simulink model "PWM"  (Simulink 7.5)
settings: Solver=VariableStepDiscrete  StartTime=0.0  StopTime=1  MaxStep=0.0001  RelTol=1e-3
libraries: simulink x1, powerlib x1
settings Model: Creator=lm  LastModifiedBy=lm

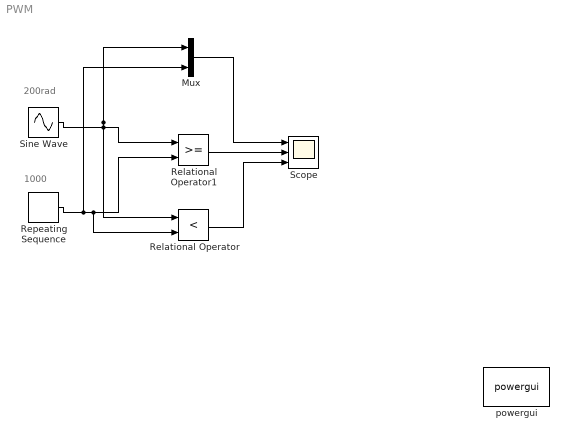
== system PWM ==
  note: 200rad
  note: 1000
  Mux : Mux  Inputs=2
  Relational Operator : RelationalOperator  Operator=<  LogicOutDataTypeMode=boolean  LogicDataType=fixdt(0, 8)  OutDataTypeStr=boolean
  Relational Operator1 : RelationalOperator  LogicOutDataTypeMode=boolean  LogicDataType=fixdt(0, 8)  OutDataTypeStr=boolean
  Repeating Sequence : simulink/Sources/Repeating Sequence  SystemSampleTime=-1  rep_seq_t=[0 0.002]  rep_seq_y=[-1 1]
  Scope : Scope  NumInputPorts=3
      settings: TimeRange=5  YMin=0~-5~-5  YMax=1~5~5
  Sine Wave : Sin  Amplitude=0.8  Bias=0  Frequency=200  Phase=0  Samples=0.02  SampleTime=0  Offset=0
  powergui : powerlib/powergui  Priority=1  SystemSampleTime=-1  SimulationMode=Continuous  SampleTime=50e-6  frequency=60  SPID=off  DisableSnubberDevices=off  DisableRonSwitches=off  DisableVfSwitches=off  SwTol=0  Interpol=off  frequencyindice=60  echomessages=off  HookPort=off  DisplayEquations=off  FunctionMessages=off  EnableUseOfTLC=off  x0status=blocks  RestoreLinks=warning  ResistiveCurrentMeasurement=off  Ylog=off  Xlog=on  ShowGrid=off  save=off  variable=ZData  ZoomFFT=off  StartTime=0.0  cycles=1  DisplayStyle=1  FreqAxis=off  MaxFrequency=1000  frequencyindicesteady=1  display=off  methode=off
  wires:
  Sine Wave/1 -> Relational Operator1/1, Mux/1, Relational Operator/1
  Repeating Sequence/1 -> Mux/2, Relational Operator1/2, Relational Operator/2
  Mux/1 -> Scope/1
  Relational Operator1/1 -> Scope/2
  Relational Operator/1 -> Scope/3
